simulink model "untitled1"  (R2018b)
settings: Solver=VariableStepAuto  StartTime=0.0  StopTime=10.0  RelTol=1e-3
settings Model: Creator=Administrator  LastModifiedBy=Administrator

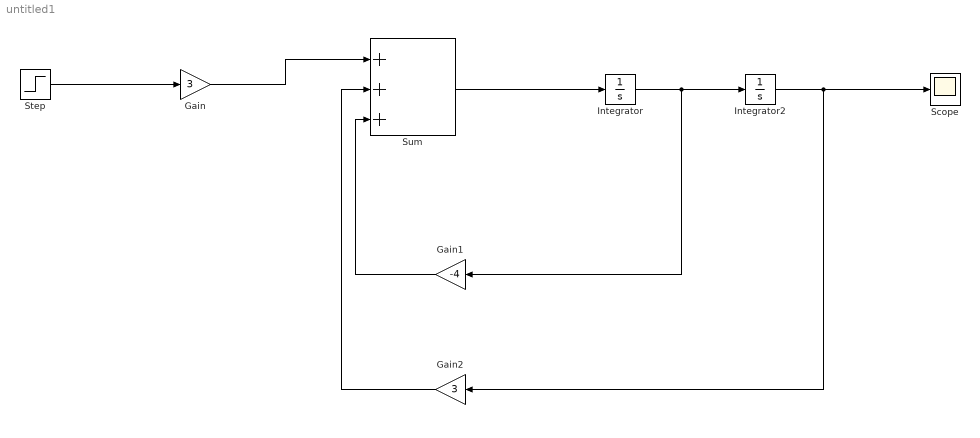
== system untitled1 ==
  Gain : Gain  Gain=3
  Gain1 : Gain  Gain=-4
  Gain2 : Gain  Gain=3
  Integrator : Integrator
  Integrator2 : Integrator
  Scope : Scope
  Step : Step  SampleTime=0
  Sum : Sum  Inputs=|+++
  wires:
  Step/1 -> Gain/1
  Gain/1 -> Sum/1
  Sum/1 -> Integrator/1
  Integrator/1 -> Gain1/1, Integrator2/1
  Integrator2/1 -> Gain2/1, Scope/1
  Gain1/1 -> Sum/3
  Gain2/1 -> Sum/2
